simulink model "on_off_control_oven"  (R2018b)
settings: Solver=VariableStepAuto  StartTime=0.0  StopTime=1000  RelTol=1e-3
settings Model: Creator=root  LastModifiedBy=root

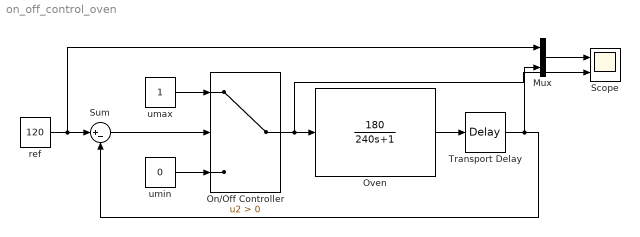
== system on_off_control_oven ==
  Mux : Mux  Inputs=2
  On/Off Controller : Switch  Criteria=u2 > Threshold
  Oven : TransferFcn  Numerator=[180]  Denominator=[240 1]
  Scope : Scope  NumInputPorts=2
  Sum : Sum  Inputs=|+-
  Transport Delay : TransportDelay  DelayTime=30
  ref : Constant  Value=120
  "umax " : Constant
  umin : Constant  Value=0
  wires:
  Oven/1 -> Transport Delay/1
  Sum/1 -> On/Off Controller/2
  "umax "/1 -> On/Off Controller/1
  ref/1 -> Mux/1, Sum/1
  umin/1 -> On/Off Controller/3
  On/Off Controller/1 -> Scope/2, Oven/1
  Mux/1 -> Scope/1
  Transport Delay/1 -> Mux/2, Sum/2
